simulink model "ModelSim"  (R2021b)
settings: Solver=VariableStepAuto  StartTime=0.0  StopTime=10000  MaxStep=0.01  RelTol=1e-3
undefined symbols (not defined in the file or in its folder): A_matrix_lin, B_matrix_lin, Bd_matrix_lin, omega_op, T_ambi_OP, Theta_1_op, Theta_2_op, U_fan_1_op, U_fan_2_op
settings Model: Creator=rasmu  LastModifiedBy=rasmu

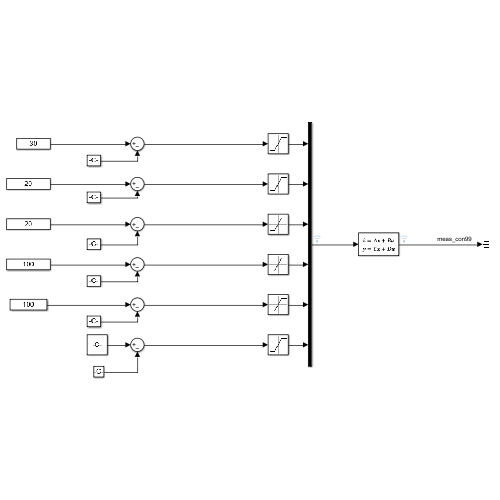
[thumbnail: Simulink's stored preview of the top-level diagram]
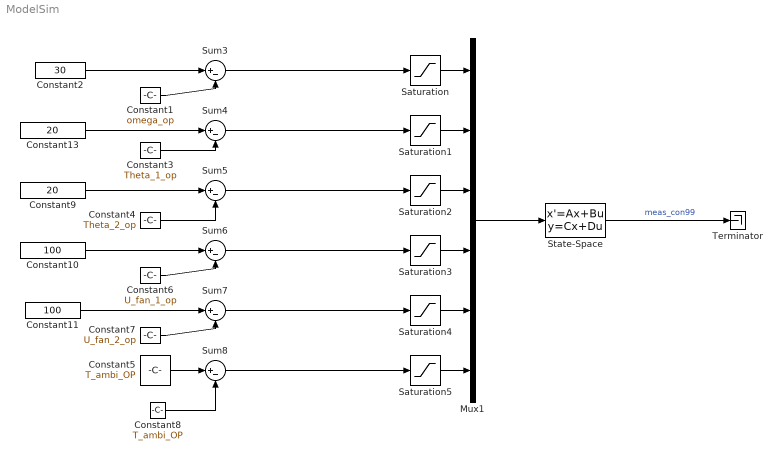
== system ModelSim ==
  Constant1 : Constant  Value=omega_op
  Constant10 : Constant  Value=100
  Constant11 : Constant  Value=100
  Constant13 : Constant  Value=20
  Constant2 : Constant  Value=30
  Constant3 : Constant  Value=Theta_1_op
  Constant4 : Constant  Value=Theta_2_op
  Constant5 : Constant  Value=T_ambi_OP
  Constant6 : Constant  Value=U_fan_1_op
  Constant7 : Constant  Value=U_fan_2_op
  Constant8 : Constant  Value=T_ambi_OP
  Constant9 : Constant  Value=20
  Mux1 : Mux  Inputs=6
  Saturation{,1..5} (6 alike) : Saturate  UpperLimit=100  LowerLimit=0
  State-Space : StateSpace  A=A_matrix_lin  B=[B_matrix_lin Bd_matrix_lin]  C=eye(11)  D=zeros(11,6)  InitialCondition=0
  Sum{3..8} (6 alike) : Sum  Inputs=|+-
  Terminator : Terminator
  wires:
  Constant4/1 -> Sum5/2
  Constant3/1 -> Sum4/2
  Constant1/1 -> Sum3/2
  Constant11/1 -> Sum7/1
  Constant13/1 -> Sum4/1
  State-Space/1 -> Terminator/1  "meas_con99"
  Constant10/1 -> Sum6/1
  Constant2/1 -> Sum3/1
  Constant5/1 -> Sum8/1
  Constant7/1 -> Sum7/2
  Mux1/1 -> State-Space/1
  Constant6/1 -> Sum6/2
  Constant8/1 -> Sum8/2
  Sum3/1 -> Saturation/1
  Sum4/1 -> Saturation1/1
  Sum5/1 -> Saturation2/1
  Sum6/1 -> Saturation3/1
  Sum7/1 -> Saturation4/1
  Sum8/1 -> Saturation5/1
  Constant9/1 -> Sum5/1
  Saturation/1 -> Mux1/1
  Saturation1/1 -> Mux1/2
  Saturation2/1 -> Mux1/3
  Saturation3/1 -> Mux1/4
  Saturation4/1 -> Mux1/5
  Saturation5/1 -> Mux1/6
